simulink model "Foster_equiv_compact_therm_network_of_IGBT_module"  (R2015a)
settings: Solver=ode45  StartTime=0.0  StopTime=10.0  RelTol=1e-3
libraries: fl_lib x20
settings Model: Creator=Caner  LastModifiedBy=Caner

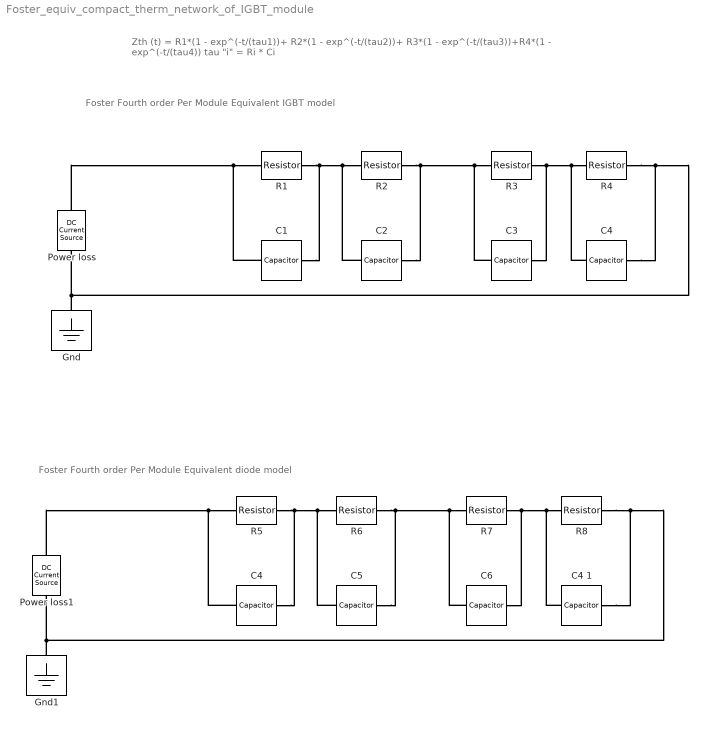
== system Foster_equiv_compact_therm_network_of_IGBT_module ==
  note: Zth (t) = R1*(1 - exp^(-t/(tau1))+ R2*(1 - exp^(-t/(tau2))+ R3*(1 - exp^(-t/(tau3))+R4*(1 - exp^(-t/(tau4))
      |
      | tau "i" = Ri * Ci
  note: Foster Fourth order Per Module Equivalent diode model
  note: Foster Fourth order Per Module Equivalent IGBT model
  C{1..6} (6 alike) : fl_lib/Electrical/Electrical Elements/Capacitor  c=1e-6 F  r=1e-6 Ohm  g=0 1/Ohm  i_specify=off  i_priority=High  i=0 A  v_specify=off  v_priority=High  v=0 V  vc_specify=off  vc_priority=High  vc=0 V
  "C4 " : fl_lib/Electrical/Electrical Elements/Capacitor  c=1e-6 F  r=1e-6 Ohm  g=0 1/Ohm  i_specify=off  i_priority=High  i=0 A  v_specify=off  v_priority=High  v=0 V  vc_specify=off  vc_priority=High  vc=0 V
  C4 1 : fl_lib/Electrical/Electrical Elements/Capacitor  c=1e-6 F  r=1e-6 Ohm  g=0 1/Ohm  i_specify=off  i_priority=High  i=0 A  v_specify=off  v_priority=High  v=0 V  vc_specify=off  vc_priority=High  vc=0 V
  Gnd : fl_lib/Electrical/Electrical Elements/Electrical Reference
  Gnd1 : fl_lib/Electrical/Electrical Elements/Electrical Reference
  Power loss : fl_lib/Electrical/Electrical Sources/DC Current Source  i0=1 A
  Power loss1 : fl_lib/Electrical/Electrical Sources/DC Current Source  i0=1 A
  R{1..8} (8 alike) : fl_lib/Electrical/Electrical Elements/Resistor  R=1 Ohm  i_specify=off  i_priority=High  i=0 A  v_specify=off  v_priority=High  v=0 V
  connections:
  Power loss/LConn1 -- C1/RConn1 -- R1/LConn1
  R1/RConn1 -- C1/LConn1 -- C2/RConn1 -- R2/LConn1
  R2/RConn1 -- C2/LConn1 -- C3/RConn1 -- R3/LConn1
  R3/RConn1 -- C3/LConn1 -- "C4 "/RConn1 -- R4/LConn1
  R4/RConn1 -- "C4 "/LConn1 -- Gnd/LConn1 -- Power loss/RConn1
  Power loss1/LConn1 -- C4/RConn1 -- R5/LConn1
  R5/RConn1 -- C4/LConn1 -- C5/RConn1 -- R6/LConn1
  R6/RConn1 -- C5/LConn1 -- C6/RConn1 -- R7/LConn1
  R7/RConn1 -- C6/LConn1 -- C4 1/RConn1 -- R8/LConn1
  Power loss1/RConn1 -- C4 1/LConn1 -- R8/RConn1 -- Gnd1/LConn1
